simulink model "test_final_sift"  (R2015a)
settings: Solver=ode45  StartTime=0.0  StopTime=10.0  RelTol=1e-3
InitFcn:
  | %% DSPBuilder Start
  | alt_dspbuilder_update_model(bdroot)
  | %% DSPBuilder End
libraries: allblocks_alteradspbuilder2 x2309
(part 5 of 27)

== system test_final_sift/sift_octave1/get_descriptor/hist_bin/Line_buffer_5x5 ==
  dataIn : Inport
  clken : Inport  Port=2
  Delay : allblocks_alteradspbuilder2/Delay  pipeline=1  pipeline_display=1  ClockPhase=1  use_ena=on  use_sclr=off  allowFloatingPointOverride=on  logOutputs=off  logFile=C:\Users\ASUS\Desktop\sift_fpga\Octave_2\tb_test_final_sift\test%5Ffinal%5Fsift_sift%5Foctave1_get%5Fdescriptor_hist%5Fbin_Line%5Fbuffer%5F5x5_Delay.fixedpointlog  use_init=off  reset_value=1
  Delay1 : allblocks_alteradspbuilder2/Delay  pipeline=1  pipeline_display=1  ClockPhase=1  use_ena=on  use_sclr=off  allowFloatingPointOverride=on  logOutputs=off  logFile=C:\Users\ASUS\Desktop\sift_fpga\Octave_2\tb_test_final_sift\test%5Ffinal%5Fsift_sift%5Foctave1_get%5Fdescriptor_hist%5Fbin_Line%5Fbuffer%5F5x5_Delay1.fixedpointlog  use_init=off  reset_value=1
  Delay10 : allblocks_alteradspbuilder2/Delay  pipeline=1  pipeline_display=1  ClockPhase=1  use_ena=on  use_sclr=off  allowFloatingPointOverride=on  logOutputs=off  logFile=C:\Users\ASUS\Desktop\sift_fpga\Octave_2\tb_test_final_sift\test%5Ffinal%5Fsift_sift%5Foctave1_get%5Fdescriptor_hist%5Fbin_Line%5Fbuffer%5F5x5_Delay10.fixedpointlog  use_init=off  reset_value=1
  Delay11 : allblocks_alteradspbuilder2/Delay  pipeline=1  pipeline_display=1  ClockPhase=1  use_ena=on  use_sclr=off  allowFloatingPointOverride=on  logOutputs=off  logFile=C:\Users\ASUS\Desktop\sift_fpga\Octave_2\tb_test_final_sift\test%5Ffinal%5Fsift_sift%5Foctave1_get%5Fdescriptor_hist%5Fbin_Line%5Fbuffer%5F5x5_Delay11.fixedpointlog  use_init=off  reset_value=1
  Delay12 : allblocks_alteradspbuilder2/Delay  pipeline=1  pipeline_display=1  ClockPhase=1  use_ena=on  use_sclr=off  allowFloatingPointOverride=on  logOutputs=off  logFile=C:\Users\ASUS\Desktop\sift_fpga\Octave_2\tb_test_final_sift\test%5Ffinal%5Fsift_sift%5Foctave1_get%5Fdescriptor_hist%5Fbin_Line%5Fbuffer%5F5x5_Delay12.fixedpointlog  use_init=off  reset_value=1
  Delay13 : allblocks_alteradspbuilder2/Delay  pipeline=1  pipeline_display=1  ClockPhase=1  use_ena=on  use_sclr=off  allowFloatingPointOverride=on  logOutputs=off  logFile=C:\Users\ASUS\Desktop\sift_fpga\Octave_2\tb_test_final_sift\test%5Ffinal%5Fsift_sift%5Foctave1_get%5Fdescriptor_hist%5Fbin_Line%5Fbuffer%5F5x5_Delay13.fixedpointlog  use_init=off  reset_value=1
  Delay14 : allblocks_alteradspbuilder2/Delay  pipeline=1  pipeline_display=1  ClockPhase=1  use_ena=on  use_sclr=off  allowFloatingPointOverride=on  logOutputs=off  logFile=C:\Users\ASUS\Desktop\sift_fpga\Octave_2\tb_test_final_sift\test%5Ffinal%5Fsift_sift%5Foctave1_get%5Fdescriptor_hist%5Fbin_Line%5Fbuffer%5F5x5_Delay14.fixedpointlog  use_init=off  reset_value=1
  Delay15 : allblocks_alteradspbuilder2/Delay  pipeline=1  pipeline_display=1  ClockPhase=1  use_ena=on  use_sclr=off  allowFloatingPointOverride=on  logOutputs=off  logFile=C:\Users\ASUS\Desktop\sift_fpga\Octave_2\tb_test_final_sift\test%5Ffinal%5Fsift_sift%5Foctave1_get%5Fdescriptor_hist%5Fbin_Line%5Fbuffer%5F5x5_Delay15.fixedpointlog  use_init=off  reset_value=1
  Delay16 : allblocks_alteradspbuilder2/Delay  pipeline=1  pipeline_display=1  ClockPhase=1  use_ena=on  use_sclr=off  allowFloatingPointOverride=on  logOutputs=off  logFile=C:\Users\ASUS\Desktop\sift_fpga\Octave_2\tb_test_final_sift\test%5Ffinal%5Fsift_sift%5Foctave1_get%5Fdescriptor_hist%5Fbin_Line%5Fbuffer%5F5x5_Delay16.fixedpointlog  use_init=off  reset_value=1
  Delay17 : allblocks_alteradspbuilder2/Delay  pipeline=1  pipeline_display=1  ClockPhase=1  use_ena=on  use_sclr=off  allowFloatingPointOverride=on  logOutputs=off  logFile=C:\Users\ASUS\Desktop\sift_fpga\Octave_2\tb_test_final_sift\test%5Ffinal%5Fsift_sift%5Foctave1_get%5Fdescriptor_hist%5Fbin_Line%5Fbuffer%5F5x5_Delay17.fixedpointlog  use_init=off  reset_value=1
  Delay18 : allblocks_alteradspbuilder2/Delay  pipeline=1  pipeline_display=1  ClockPhase=1  use_ena=on  use_sclr=off  allowFloatingPointOverride=on  logOutputs=off  logFile=C:\Users\ASUS\Desktop\sift_fpga\Octave_2\tb_test_final_sift\test%5Ffinal%5Fsift_sift%5Foctave1_get%5Fdescriptor_hist%5Fbin_Line%5Fbuffer%5F5x5_Delay18.fixedpointlog  use_init=off  reset_value=1
  Delay19 : allblocks_alteradspbuilder2/Delay  pipeline=1  pipeline_display=1  ClockPhase=1  use_ena=on  use_sclr=off  allowFloatingPointOverride=on  logOutputs=off  logFile=C:\Users\ASUS\Desktop\sift_fpga\Octave_2\tb_test_final_sift\test%5Ffinal%5Fsift_sift%5Foctave1_get%5Fdescriptor_hist%5Fbin_Line%5Fbuffer%5F5x5_Delay19.fixedpointlog  use_init=off  reset_value=1
  Delay2 : allblocks_alteradspbuilder2/Delay  pipeline=1  pipeline_display=1  ClockPhase=1  use_ena=on  use_sclr=off  allowFloatingPointOverride=on  logOutputs=off  logFile=C:\Users\ASUS\Desktop\sift_fpga\Octave_2\tb_test_final_sift\test%5Ffinal%5Fsift_sift%5Foctave1_get%5Fdescriptor_hist%5Fbin_Line%5Fbuffer%5F5x5_Delay2.fixedpointlog  use_init=off  reset_value=1
  Delay20 : allblocks_alteradspbuilder2/Delay  pipeline=1  pipeline_display=1  ClockPhase=1  use_ena=on  use_sclr=off  allowFloatingPointOverride=on  logOutputs=off  logFile=C:\Users\ASUS\Desktop\sift_fpga\Octave_2\tb_test_final_sift\test%5Ffinal%5Fsift_sift%5Foctave1_get%5Fdescriptor_hist%5Fbin_Line%5Fbuffer%5F5x5_Delay20.fixedpointlog  use_init=off  reset_value=1
  Delay3 : allblocks_alteradspbuilder2/Delay  pipeline=1  pipeline_display=1  ClockPhase=1  use_ena=on  use_sclr=off  allowFloatingPointOverride=on  logOutputs=off  logFile=C:\Users\ASUS\Desktop\sift_fpga\Octave_2\tb_test_final_sift\test%5Ffinal%5Fsift_sift%5Foctave1_get%5Fdescriptor_hist%5Fbin_Line%5Fbuffer%5F5x5_Delay3.fixedpointlog  use_init=off  reset_value=1
  Delay4 : allblocks_alteradspbuilder2/Delay  pipeline=1  pipeline_display=1  ClockPhase=1  use_ena=on  use_sclr=off  allowFloatingPointOverride=on  logOutputs=off  logFile=C:\Users\ASUS\Desktop\sift_fpga\Octave_2\tb_test_final_sift\test%5Ffinal%5Fsift_sift%5Foctave1_get%5Fdescriptor_hist%5Fbin_Line%5Fbuffer%5F5x5_Delay4.fixedpointlog  use_init=off  reset_value=1
  Delay5 : allblocks_alteradspbuilder2/Delay  pipeline=1  pipeline_display=1  ClockPhase=1  use_ena=on  use_sclr=off  allowFloatingPointOverride=on  logOutputs=off  logFile=C:\Users\ASUS\Desktop\sift_fpga\Octave_2\tb_test_final_sift\test%5Ffinal%5Fsift_sift%5Foctave1_get%5Fdescriptor_hist%5Fbin_Line%5Fbuffer%5F5x5_Delay5.fixedpointlog  use_init=off  reset_value=1
  Delay6 : allblocks_alteradspbuilder2/Delay  pipeline=1  pipeline_display=1  ClockPhase=1  use_ena=on  use_sclr=off  allowFloatingPointOverride=on  logOutputs=off  logFile=C:\Users\ASUS\Desktop\sift_fpga\Octave_2\tb_test_final_sift\test%5Ffinal%5Fsift_sift%5Foctave1_get%5Fdescriptor_hist%5Fbin_Line%5Fbuffer%5F5x5_Delay6.fixedpointlog  use_init=off  reset_value=1
  Delay7 : allblocks_alteradspbuilder2/Delay  pipeline=1  pipeline_display=1  ClockPhase=1  use_ena=on  use_sclr=off  allowFloatingPointOverride=on  logOutputs=off  logFile=C:\Users\ASUS\Desktop\sift_fpga\Octave_2\tb_test_final_sift\test%5Ffinal%5Fsift_sift%5Foctave1_get%5Fdescriptor_hist%5Fbin_Line%5Fbuffer%5F5x5_Delay7.fixedpointlog  use_init=off  reset_value=1
  Delay8 : allblocks_alteradspbuilder2/Delay  pipeline=1  pipeline_display=1  ClockPhase=1  use_ena=on  use_sclr=off  allowFloatingPointOverride=on  logOutputs=off  logFile=C:\Users\ASUS\Desktop\sift_fpga\Octave_2\tb_test_final_sift\test%5Ffinal%5Fsift_sift%5Foctave1_get%5Fdescriptor_hist%5Fbin_Line%5Fbuffer%5F5x5_Delay8.fixedpointlog  use_init=off  reset_value=1
  Delay9 : allblocks_alteradspbuilder2/Delay  pipeline=1  pipeline_display=1  ClockPhase=1  use_ena=on  use_sclr=off  allowFloatingPointOverride=on  logOutputs=off  logFile=C:\Users\ASUS\Desktop\sift_fpga\Octave_2\tb_test_final_sift\test%5Ffinal%5Fsift_sift%5Foctave1_get%5Fdescriptor_hist%5Fbin_Line%5Fbuffer%5F5x5_Delay9.fixedpointlog  use_init=off  reset_value=1
  Memory Delay : allblocks_alteradspbuilder2/Memory Delay  BusType=Unsigned Integer  bwl=10  bwr=0  pipeline=636  pipeline_display=636  ram_type=AUTO  use_ena=on  use_sclr=off  allowFloatingPointOverride=on  logOutputs=off  logFile=C:\Users\ASUS\Desktop\sift_fpga\Octave_2\tb_test_final_sift\test%5Ffinal%5Fsift_sift%5Foctave1_get%5Fdescriptor_hist%5Fbin_Line%5Fbuffer%5F5x5_Memory+Delay.fixedpointlog
  Memory Delay1 : allblocks_alteradspbuilder2/Memory Delay  BusType=Unsigned Integer  bwl=10  bwr=0  pipeline=636  pipeline_display=636  ram_type=AUTO  use_ena=on  use_sclr=off  allowFloatingPointOverride=on  logOutputs=off  logFile=C:\Users\ASUS\Desktop\sift_fpga\Octave_2\tb_test_final_sift\test%5Ffinal%5Fsift_sift%5Foctave1_get%5Fdescriptor_hist%5Fbin_Line%5Fbuffer%5F5x5_Memory+Delay1.fixedpointlog
  Memory Delay2 : allblocks_alteradspbuilder2/Memory Delay  BusType=Unsigned Integer  bwl=10  bwr=0  pipeline=636  pipeline_display=636  ram_type=AUTO  use_ena=on  use_sclr=off  allowFloatingPointOverride=on  logOutputs=off  logFile=C:\Users\ASUS\Desktop\sift_fpga\Octave_2\tb_test_final_sift\test%5Ffinal%5Fsift_sift%5Foctave1_get%5Fdescriptor_hist%5Fbin_Line%5Fbuffer%5F5x5_Memory+Delay2.fixedpointlog
  Memory Delay3 : allblocks_alteradspbuilder2/Memory Delay  BusType=Unsigned Integer  bwl=10  bwr=0  pipeline=636  pipeline_display=636  ram_type=AUTO  use_ena=on  use_sclr=off  allowFloatingPointOverride=on  logOutputs=off  logFile=C:\Users\ASUS\Desktop\sift_fpga\Octave_2\tb_test_final_sift\test%5Ffinal%5Fsift_sift%5Foctave1_get%5Fdescriptor_hist%5Fbin_Line%5Fbuffer%5F5x5_Memory+Delay3.fixedpointlog
  Out00 : Outport
  Out01 : Outport  Port=2
  Out02 : Outport  Port=3
  Out03 : Outport  Port=4
  Out04 : Outport  Port=5
  Out10 : Outport  Port=6
  Out11 : Outport  Port=7
  Out12 : Outport  Port=8
  Out13 : Outport  Port=9
  Out14 : Outport  Port=10
  Out20 : Outport  Port=11
  Out21 : Outport  Port=12
  Out22 : Outport  Port=13
  Out23 : Outport  Port=14
  Out24 : Outport  Port=15
  Out30 : Outport  Port=16
  Out31 : Outport  Port=17
  Out32 : Outport  Port=18
  Out33 : Outport  Port=19
  Out34 : Outport  Port=20
  Out40 : Outport  Port=21
  Out41 : Outport  Port=22
  Out42 : Outport  Port=23
  Out43 : Outport  Port=24
  Out44 : Outport  Port=25
  wires:
  [clken] -> Delay11/2
  Delay11/1 -> [data_23], Delay12/1
  [clken] -> Delay12/2
  [clken] -> Delay10/2
  Delay8/1 -> Memory Delay1/1, [data_14]
  [clken] -> Memory Delay1/2
  Delay9/1 -> [data_21], Delay10/1
  Memory Delay1/1 -> [data_20], Delay9/1
  Delay10/1 -> [data_22], Delay11/1
  [clken] -> Delay9/2
  [clken] -> Delay4/2
  [data_03] -> Out03/1
  [data_04] -> Out04/1
  [data_02] -> Out02/1
  Delay/1 -> [data_00], Delay1/1
  [data_32] -> Out32/1
  [data_44] -> Out44/1
  [data_31] -> Out31/1
  [data_40] -> Out40/1
  [data_34] -> Out34/1
  [data_30] -> Out30/1
  [data_33] -> Out33/1
  [data_43] -> Out43/1
  [data_42] -> Out42/1
  [data_41] -> Out41/1
  [clken] -> Delay1/2
  [clken] -> Delay/2
  [data_in] -> Delay/1
  [clken] -> Delay2/2
  Delay2/1 -> [data_02], Delay3/1
  Delay1/1 -> [data_01], Delay2/1
  [clken] -> Delay3/2
  [data_01] -> Out01/1
  clken/1 -> [clken]
  [data_00] -> Out00/1
  [data_21] -> Out21/1
  [data_20] -> Out20/1
  [data_23] -> Out23/1
  [data_22] -> Out22/1
  [data_24] -> Out24/1
  dataIn/1 -> [data_in]
  [data_10] -> Out10/1
  [data_11] -> Out11/1
  [data_12] -> Out12/1
  [data_13] -> Out13/1
  [data_14] -> Out14/1
  Delay4/1 -> Memory Delay/1, [data_04]
  [clken] -> Memory Delay/2
  Delay12/1 -> [data_24], Memory Delay2/1
  [clken] -> Memory Delay2/2
  Memory Delay2/1 -> [data_30], Delay16/1
  [clken] -> Delay16/2
  [clken] -> Delay14/2
  [clken] -> Delay15/2
  [clken] -> Memory Delay3/2
  Delay17/1 -> [data_32], Delay18/1
  Delay18/1 -> [data_33], Delay19/1
  Memory Delay3/1 -> [data_40], Delay20/1
  [clken] -> Delay20/2
  [clken] -> Delay19/2
  Delay13/1 -> [data_42], Delay14/1
  Delay19/1 -> Memory Delay3/1, [data_34]
  Delay14/1 -> [data_43], Delay15/1
  Delay15/1 -> [data_44]
  [clken] -> Delay17/2
  [clken] -> Delay18/2
  [clken] -> Delay13/2
  Delay16/1 -> [data_31], Delay17/1
  Delay20/1 -> [data_41], Delay13/1
  Memory Delay/1 -> [data_10], Delay5/1
  [clken] -> Delay7/2
  [clken] -> Delay6/2
  Delay5/1 -> [data_11], Delay6/1
  [clken] -> Delay8/2
  [clken] -> Delay5/2
  Delay7/1 -> [data_13], Delay8/1
  Delay6/1 -> [data_12], Delay7/1
  Delay3/1 -> [data_03], Delay4/1

== system test_final_sift/sift_octave1/get_descriptor/hist_bin/Line_buffer_5x5_1 ==
  dataIn : Inport
  clken : Inport  Port=2
  Delay : allblocks_alteradspbuilder2/Delay  pipeline=1  pipeline_display=1  ClockPhase=1  use_ena=on  use_sclr=off  allowFloatingPointOverride=on  logOutputs=off  logFile=C:\Users\ASUS\Desktop\sift_fpga\Octave_2\tb_test_final_sift\test%5Ffinal%5Fsift_sift%5Foctave1_get%5Fdescriptor_hist%5Fbin_Line%5Fbuffer%5F5x5%5F1_Delay.fixedpointlog  use_init=off  reset_value=1
  Delay1 : allblocks_alteradspbuilder2/Delay  pipeline=1  pipeline_display=1  ClockPhase=1  use_ena=on  use_sclr=off  allowFloatingPointOverride=on  logOutputs=off  logFile=C:\Users\ASUS\Desktop\sift_fpga\Octave_2\tb_test_final_sift\test%5Ffinal%5Fsift_sift%5Foctave1_get%5Fdescriptor_hist%5Fbin_Line%5Fbuffer%5F5x5%5F1_Delay1.fixedpointlog  use_init=off  reset_value=1
  Delay10 : allblocks_alteradspbuilder2/Delay  pipeline=1  pipeline_display=1  ClockPhase=1  use_ena=on  use_sclr=off  allowFloatingPointOverride=on  logOutputs=off  logFile=C:\Users\ASUS\Desktop\sift_fpga\Octave_2\tb_test_final_sift\test%5Ffinal%5Fsift_sift%5Foctave1_get%5Fdescriptor_hist%5Fbin_Line%5Fbuffer%5F5x5%5F1_Delay10.fixedpointlog  use_init=off  reset_value=1
  Delay11 : allblocks_alteradspbuilder2/Delay  pipeline=1  pipeline_display=1  ClockPhase=1  use_ena=on  use_sclr=off  allowFloatingPointOverride=on  logOutputs=off  logFile=C:\Users\ASUS\Desktop\sift_fpga\Octave_2\tb_test_final_sift\test%5Ffinal%5Fsift_sift%5Foctave1_get%5Fdescriptor_hist%5Fbin_Line%5Fbuffer%5F5x5%5F1_Delay11.fixedpointlog  use_init=off  reset_value=1
  Delay12 : allblocks_alteradspbuilder2/Delay  pipeline=1  pipeline_display=1  ClockPhase=1  use_ena=on  use_sclr=off  allowFloatingPointOverride=on  logOutputs=off  logFile=C:\Users\ASUS\Desktop\sift_fpga\Octave_2\tb_test_final_sift\test%5Ffinal%5Fsift_sift%5Foctave1_get%5Fdescriptor_hist%5Fbin_Line%5Fbuffer%5F5x5%5F1_Delay12.fixedpointlog  use_init=off  reset_value=1
  Delay13 : allblocks_alteradspbuilder2/Delay  pipeline=1  pipeline_display=1  ClockPhase=1  use_ena=on  use_sclr=off  allowFloatingPointOverride=on  logOutputs=off  logFile=C:\Users\ASUS\Desktop\sift_fpga\Octave_2\tb_test_final_sift\test%5Ffinal%5Fsift_sift%5Foctave1_get%5Fdescriptor_hist%5Fbin_Line%5Fbuffer%5F5x5%5F1_Delay13.fixedpointlog  use_init=off  reset_value=1
  Delay14 : allblocks_alteradspbuilder2/Delay  pipeline=1  pipeline_display=1  ClockPhase=1  use_ena=on  use_sclr=off  allowFloatingPointOverride=on  logOutputs=off  logFile=C:\Users\ASUS\Desktop\sift_fpga\Octave_2\tb_test_final_sift\test%5Ffinal%5Fsift_sift%5Foctave1_get%5Fdescriptor_hist%5Fbin_Line%5Fbuffer%5F5x5%5F1_Delay14.fixedpointlog  use_init=off  reset_value=1
  Delay15 : allblocks_alteradspbuilder2/Delay  pipeline=1  pipeline_display=1  ClockPhase=1  use_ena=on  use_sclr=off  allowFloatingPointOverride=on  logOutputs=off  logFile=C:\Users\ASUS\Desktop\sift_fpga\Octave_2\tb_test_final_sift\test%5Ffinal%5Fsift_sift%5Foctave1_get%5Fdescriptor_hist%5Fbin_Line%5Fbuffer%5F5x5%5F1_Delay15.fixedpointlog  use_init=off  reset_value=1
  Delay16 : allblocks_alteradspbuilder2/Delay  pipeline=1  pipeline_display=1  ClockPhase=1  use_ena=on  use_sclr=off  allowFloatingPointOverride=on  logOutputs=off  logFile=C:\Users\ASUS\Desktop\sift_fpga\Octave_2\tb_test_final_sift\test%5Ffinal%5Fsift_sift%5Foctave1_get%5Fdescriptor_hist%5Fbin_Line%5Fbuffer%5F5x5%5F1_Delay16.fixedpointlog  use_init=off  reset_value=1
  Delay17 : allblocks_alteradspbuilder2/Delay  pipeline=1  pipeline_display=1  ClockPhase=1  use_ena=on  use_sclr=off  allowFloatingPointOverride=on  logOutputs=off  logFile=C:\Users\ASUS\Desktop\sift_fpga\Octave_2\tb_test_final_sift\test%5Ffinal%5Fsift_sift%5Foctave1_get%5Fdescriptor_hist%5Fbin_Line%5Fbuffer%5F5x5%5F1_Delay17.fixedpointlog  use_init=off  reset_value=1
  Delay18 : allblocks_alteradspbuilder2/Delay  pipeline=1  pipeline_display=1  ClockPhase=1  use_ena=on  use_sclr=off  allowFloatingPointOverride=on  logOutputs=off  logFile=C:\Users\ASUS\Desktop\sift_fpga\Octave_2\tb_test_final_sift\test%5Ffinal%5Fsift_sift%5Foctave1_get%5Fdescriptor_hist%5Fbin_Line%5Fbuffer%5F5x5%5F1_Delay18.fixedpointlog  use_init=off  reset_value=1
  Delay19 : allblocks_alteradspbuilder2/Delay  pipeline=1  pipeline_display=1  ClockPhase=1  use_ena=on  use_sclr=off  allowFloatingPointOverride=on  logOutputs=off  logFile=C:\Users\ASUS\Desktop\sift_fpga\Octave_2\tb_test_final_sift\test%5Ffinal%5Fsift_sift%5Foctave1_get%5Fdescriptor_hist%5Fbin_Line%5Fbuffer%5F5x5%5F1_Delay19.fixedpointlog  use_init=off  reset_value=1
  Delay2 : allblocks_alteradspbuilder2/Delay  pipeline=1  pipeline_display=1  ClockPhase=1  use_ena=on  use_sclr=off  allowFloatingPointOverride=on  logOutputs=off  logFile=C:\Users\ASUS\Desktop\sift_fpga\Octave_2\tb_test_final_sift\test%5Ffinal%5Fsift_sift%5Foctave1_get%5Fdescriptor_hist%5Fbin_Line%5Fbuffer%5F5x5%5F1_Delay2.fixedpointlog  use_init=off  reset_value=1
  Delay20 : allblocks_alteradspbuilder2/Delay  pipeline=1  pipeline_display=1  ClockPhase=1  use_ena=on  use_sclr=off  allowFloatingPointOverride=on  logOutputs=off  logFile=C:\Users\ASUS\Desktop\sift_fpga\Octave_2\tb_test_final_sift\test%5Ffinal%5Fsift_sift%5Foctave1_get%5Fdescriptor_hist%5Fbin_Line%5Fbuffer%5F5x5%5F1_Delay20.fixedpointlog  use_init=off  reset_value=1
  Delay3 : allblocks_alteradspbuilder2/Delay  pipeline=1  pipeline_display=1  ClockPhase=1  use_ena=on  use_sclr=off  allowFloatingPointOverride=on  logOutputs=off  logFile=C:\Users\ASUS\Desktop\sift_fpga\Octave_2\tb_test_final_sift\test%5Ffinal%5Fsift_sift%5Foctave1_get%5Fdescriptor_hist%5Fbin_Line%5Fbuffer%5F5x5%5F1_Delay3.fixedpointlog  use_init=off  reset_value=1
  Delay4 : allblocks_alteradspbuilder2/Delay  pipeline=1  pipeline_display=1  ClockPhase=1  use_ena=on  use_sclr=off  allowFloatingPointOverride=on  logOutputs=off  logFile=C:\Users\ASUS\Desktop\sift_fpga\Octave_2\tb_test_final_sift\test%5Ffinal%5Fsift_sift%5Foctave1_get%5Fdescriptor_hist%5Fbin_Line%5Fbuffer%5F5x5%5F1_Delay4.fixedpointlog  use_init=off  reset_value=1
  Delay5 : allblocks_alteradspbuilder2/Delay  pipeline=1  pipeline_display=1  ClockPhase=1  use_ena=on  use_sclr=off  allowFloatingPointOverride=on  logOutputs=off  logFile=C:\Users\ASUS\Desktop\sift_fpga\Octave_2\tb_test_final_sift\test%5Ffinal%5Fsift_sift%5Foctave1_get%5Fdescriptor_hist%5Fbin_Line%5Fbuffer%5F5x5%5F1_Delay5.fixedpointlog  use_init=off  reset_value=1
  Delay6 : allblocks_alteradspbuilder2/Delay  pipeline=1  pipeline_display=1  ClockPhase=1  use_ena=on  use_sclr=off  allowFloatingPointOverride=on  logOutputs=off  logFile=C:\Users\ASUS\Desktop\sift_fpga\Octave_2\tb_test_final_sift\test%5Ffinal%5Fsift_sift%5Foctave1_get%5Fdescriptor_hist%5Fbin_Line%5Fbuffer%5F5x5%5F1_Delay6.fixedpointlog  use_init=off  reset_value=1
  Delay7 : allblocks_alteradspbuilder2/Delay  pipeline=1  pipeline_display=1  ClockPhase=1  use_ena=on  use_sclr=off  allowFloatingPointOverride=on  logOutputs=off  logFile=C:\Users\ASUS\Desktop\sift_fpga\Octave_2\tb_test_final_sift\test%5Ffinal%5Fsift_sift%5Foctave1_get%5Fdescriptor_hist%5Fbin_Line%5Fbuffer%5F5x5%5F1_Delay7.fixedpointlog  use_init=off  reset_value=1
  Delay8 : allblocks_alteradspbuilder2/Delay  pipeline=1  pipeline_display=1  ClockPhase=1  use_ena=on  use_sclr=off  allowFloatingPointOverride=on  logOutputs=off  logFile=C:\Users\ASUS\Desktop\sift_fpga\Octave_2\tb_test_final_sift\test%5Ffinal%5Fsift_sift%5Foctave1_get%5Fdescriptor_hist%5Fbin_Line%5Fbuffer%5F5x5%5F1_Delay8.fixedpointlog  use_init=off  reset_value=1
  Delay9 : allblocks_alteradspbuilder2/Delay  pipeline=1  pipeline_display=1  ClockPhase=1  use_ena=on  use_sclr=off  allowFloatingPointOverride=on  logOutputs=off  logFile=C:\Users\ASUS\Desktop\sift_fpga\Octave_2\tb_test_final_sift\test%5Ffinal%5Fsift_sift%5Foctave1_get%5Fdescriptor_hist%5Fbin_Line%5Fbuffer%5F5x5%5F1_Delay9.fixedpointlog  use_init=off  reset_value=1
  Memory Delay : allblocks_alteradspbuilder2/Memory Delay  BusType=Unsigned Integer  bwl=8  bwr=0  pipeline=636  pipeline_display=636  ram_type=AUTO  use_ena=on  use_sclr=off  allowFloatingPointOverride=on  logOutputs=off  logFile=C:\Users\ASUS\Desktop\sift_fpga\Octave_2\tb_test_final_sift\test%5Ffinal%5Fsift_sift%5Foctave1_get%5Fdescriptor_hist%5Fbin_Line%5Fbuffer%5F5x5%5F1_Memory+Delay.fixedpointlog
  Memory Delay1 : allblocks_alteradspbuilder2/Memory Delay  BusType=Unsigned Integer  bwl=8  bwr=0  pipeline=636  pipeline_display=636  ram_type=AUTO  use_ena=on  use_sclr=off  allowFloatingPointOverride=on  logOutputs=off  logFile=C:\Users\ASUS\Desktop\sift_fpga\Octave_2\tb_test_final_sift\test%5Ffinal%5Fsift_sift%5Foctave1_get%5Fdescriptor_hist%5Fbin_Line%5Fbuffer%5F5x5%5F1_Memory+Delay1.fixedpointlog
  Memory Delay2 : allblocks_alteradspbuilder2/Memory Delay  BusType=Unsigned Integer  bwl=8  bwr=0  pipeline=636  pipeline_display=636  ram_type=AUTO  use_ena=on  use_sclr=off  allowFloatingPointOverride=on  logOutputs=off  logFile=C:\Users\ASUS\Desktop\sift_fpga\Octave_2\tb_test_final_sift\test%5Ffinal%5Fsift_sift%5Foctave1_get%5Fdescriptor_hist%5Fbin_Line%5Fbuffer%5F5x5%5F1_Memory+Delay2.fixedpointlog
  Memory Delay3 : allblocks_alteradspbuilder2/Memory Delay  BusType=Unsigned Integer  bwl=8  bwr=0  pipeline=636  pipeline_display=636  ram_type=AUTO  use_ena=on  use_sclr=off  allowFloatingPointOverride=on  logOutputs=off  logFile=C:\Users\ASUS\Desktop\sift_fpga\Octave_2\tb_test_final_sift\test%5Ffinal%5Fsift_sift%5Foctave1_get%5Fdescriptor_hist%5Fbin_Line%5Fbuffer%5F5x5%5F1_Memory+Delay3.fixedpointlog
  Out00 : Outport
  Out01 : Outport  Port=2
  Out02 : Outport  Port=3
  Out03 : Outport  Port=4
  Out04 : Outport  Port=5
  Out10 : Outport  Port=6
  Out11 : Outport  Port=7
  Out12 : Outport  Port=8
  Out13 : Outport  Port=9
  Out14 : Outport  Port=10
  Out20 : Outport  Port=11
  Out21 : Outport  Port=12
  Out22 : Outport  Port=13
  Out23 : Outport  Port=14
  Out24 : Outport  Port=15
  Out30 : Outport  Port=16
  Out31 : Outport  Port=17
  Out32 : Outport  Port=18
  Out33 : Outport  Port=19
  Out34 : Outport  Port=20
  Out40 : Outport  Port=21
  Out41 : Outport  Port=22
  Out42 : Outport  Port=23
  Out43 : Outport  Port=24
  Out44 : Outport  Port=25
  wires:
  [clken] -> Delay11/2
  Delay11/1 -> [data_23], Delay12/1
  [clken] -> Delay12/2
  [clken] -> Delay10/2
  Delay8/1 -> Memory Delay1/1, [data_14]
  [clken] -> Memory Delay1/2
  Delay9/1 -> [data_21], Delay10/1
  Memory Delay1/1 -> [data_20], Delay9/1
  Delay10/1 -> [data_22], Delay11/1
  [clken] -> Delay9/2
  [clken] -> Delay4/2
  [data_03] -> Out03/1
  [data_04] -> Out04/1
  [data_02] -> Out02/1
  Delay/1 -> [data_00], Delay1/1
  [data_32] -> Out32/1
  [data_44] -> Out44/1
  [data_31] -> Out31/1
  [data_40] -> Out40/1
  [data_34] -> Out34/1
  [data_30] -> Out30/1
  [data_33] -> Out33/1
  [data_43] -> Out43/1
  [data_42] -> Out42/1
  [data_41] -> Out41/1
  [clken] -> Delay1/2
  [clken] -> Delay/2
  [data_in] -> Delay/1
  [clken] -> Delay2/2
  Delay2/1 -> [data_02], Delay3/1
  Delay1/1 -> [data_01], Delay2/1
  [clken] -> Delay3/2
  [data_01] -> Out01/1
  clken/1 -> [clken]
  [data_00] -> Out00/1
  [data_21] -> Out21/1
  [data_20] -> Out20/1
  [data_23] -> Out23/1
  [data_22] -> Out22/1
  [data_24] -> Out24/1
  dataIn/1 -> [data_in]
  [data_10] -> Out10/1
  [data_11] -> Out11/1
  [data_12] -> Out12/1
  [data_13] -> Out13/1
  [data_14] -> Out14/1
  Delay4/1 -> Memory Delay/1, [data_04]
  [clken] -> Memory Delay/2
  Delay12/1 -> [data_24], Memory Delay2/1
  [clken] -> Memory Delay2/2
  Memory Delay2/1 -> [data_30], Delay16/1
  [clken] -> Delay16/2
  [clken] -> Delay14/2
  [clken] -> Delay15/2
  [clken] -> Memory Delay3/2
  Delay17/1 -> [data_32], Delay18/1
  Delay18/1 -> [data_33], Delay19/1
  Memory Delay3/1 -> [data_40], Delay20/1
  [clken] -> Delay20/2
  [clken] -> Delay19/2
  Delay13/1 -> [data_42], Delay14/1
  Delay19/1 -> Memory Delay3/1, [data_34]
  Delay14/1 -> [data_43], Delay15/1
  Delay15/1 -> [data_44]
  [clken] -> Delay17/2
  [clken] -> Delay18/2
  [clken] -> Delay13/2
  Delay16/1 -> [data_31], Delay17/1
  Delay20/1 -> [data_41], Delay13/1
  Memory Delay/1 -> [data_10], Delay5/1
  [clken] -> Delay7/2
  [clken] -> Delay6/2
  Delay5/1 -> [data_11], Delay6/1
  [clken] -> Delay8/2
  [clken] -> Delay5/2
  Delay7/1 -> [data_13], Delay8/1
  Delay6/1 -> [data_12], Delay7/1
  Delay3/1 -> [data_03], Delay4/1

== system test_final_sift/sift_octave1/get_descriptor/hist_bin/Subsystem ==
  hist_in_bin1 : Inport
  hist_in_bin2 : Inport  Port=2
  hist_in_bin3 : Inport  Port=3
  hist_in_bin4 : Inport  Port=4
  hist_in_bin5 : Inport  Port=5
  hist_in_bin6 : Inport  Port=6
  hist_in_bin7 : Inport  Port=7
  hist_in_bin8 : Inport  Port=8
  Comparator1 : allblocks_alteradspbuilder2/Comparator  direction=a < b  pipeline_display=0  allowFloatingPointOverride=on  logOutputs=off  logFile=C:\Users\ASUS\Desktop\sift_fpga\Octave_2\tb_test_final_sift\test%5Ffinal%5Fsift_sift%5Foctave1_get%5Fdescriptor_hist%5Fbin_Subsystem_Comparator1.fixedpointlog
  Comparator10 : allblocks_alteradspbuilder2/Comparator  direction=a < b  pipeline_display=0  allowFloatingPointOverride=on  logOutputs=off  logFile=C:\Users\ASUS\Desktop\sift_fpga\Octave_2\tb_test_final_sift\test%5Ffinal%5Fsift_sift%5Foctave1_get%5Fdescriptor_hist%5Fbin_Subsystem_Comparator10.fixedpointlog
  Comparator11 : allblocks_alteradspbuilder2/Comparator  direction=a < b  pipeline_display=0  allowFloatingPointOverride=on  logOutputs=off  logFile=C:\Users\ASUS\Desktop\sift_fpga\Octave_2\tb_test_final_sift\test%5Ffinal%5Fsift_sift%5Foctave1_get%5Fdescriptor_hist%5Fbin_Subsystem_Comparator11.fixedpointlog
  Comparator12 : allblocks_alteradspbuilder2/Comparator  direction=a < b  pipeline_display=0  allowFloatingPointOverride=on  logOutputs=off  logFile=C:\Users\ASUS\Desktop\sift_fpga\Octave_2\tb_test_final_sift\test%5Ffinal%5Fsift_sift%5Foctave1_get%5Fdescriptor_hist%5Fbin_Subsystem_Comparator12.fixedpointlog
  Comparator13 : allblocks_alteradspbuilder2/Comparator  direction=a < b  pipeline_display=0  allowFloatingPointOverride=on  logOutputs=off  logFile=C:\Users\ASUS\Desktop\sift_fpga\Octave_2\tb_test_final_sift\test%5Ffinal%5Fsift_sift%5Foctave1_get%5Fdescriptor_hist%5Fbin_Subsystem_Comparator13.fixedpointlog
  Comparator14 : allblocks_alteradspbuilder2/Comparator  direction=a < b  pipeline_display=0  allowFloatingPointOverride=on  logOutputs=off  logFile=C:\Users\ASUS\Desktop\sift_fpga\Octave_2\tb_test_final_sift\test%5Ffinal%5Fsift_sift%5Foctave1_get%5Fdescriptor_hist%5Fbin_Subsystem_Comparator14.fixedpointlog
  Comparator19 : allblocks_alteradspbuilder2/Comparator  direction=a < b  pipeline_display=0  allowFloatingPointOverride=on  logOutputs=off  logFile=C:\Users\ASUS\Desktop\sift_fpga\Octave_2\tb_test_final_sift\test%5Ffinal%5Fsift_sift%5Foctave1_get%5Fdescriptor_hist%5Fbin_Subsystem_Comparator19.fixedpointlog
  Comparator2 : allblocks_alteradspbuilder2/Comparator  direction=a < b  pipeline_display=0  allowFloatingPointOverride=on  logOutputs=off  logFile=C:\Users\ASUS\Desktop\sift_fpga\Octave_2\tb_test_final_sift\test%5Ffinal%5Fsift_sift%5Foctave1_get%5Fdescriptor_hist%5Fbin_Subsystem_Comparator2.fixedpointlog
  Comparator3 : allblocks_alteradspbuilder2/Comparator  direction=a < b  pipeline_display=0  allowFloatingPointOverride=on  logOutputs=off  logFile=C:\Users\ASUS\Desktop\sift_fpga\Octave_2\tb_test_final_sift\test%5Ffinal%5Fsift_sift%5Foctave1_get%5Fdescriptor_hist%5Fbin_Subsystem_Comparator3.fixedpointlog
  Comparator4 : allblocks_alteradspbuilder2/Comparator  direction=a < b  pipeline_display=0  allowFloatingPointOverride=on  logOutputs=off  logFile=C:\Users\ASUS\Desktop\sift_fpga\Octave_2\tb_test_final_sift\test%5Ffinal%5Fsift_sift%5Foctave1_get%5Fdescriptor_hist%5Fbin_Subsystem_Comparator4.fixedpointlog
  Comparator5 : allblocks_alteradspbuilder2/Comparator  direction=a < b  pipeline_display=0  allowFloatingPointOverride=on  logOutputs=off  logFile=C:\Users\ASUS\Desktop\sift_fpga\Octave_2\tb_test_final_sift\test%5Ffinal%5Fsift_sift%5Foctave1_get%5Fdescriptor_hist%5Fbin_Subsystem_Comparator5.fixedpointlog
  Comparator6 : allblocks_alteradspbuilder2/Comparator  direction=a < b  pipeline_display=0  allowFloatingPointOverride=on  logOutputs=off  logFile=C:\Users\ASUS\Desktop\sift_fpga\Octave_2\tb_test_final_sift\test%5Ffinal%5Fsift_sift%5Foctave1_get%5Fdescriptor_hist%5Fbin_Subsystem_Comparator6.fixedpointlog
  Comparator7 : allblocks_alteradspbuilder2/Comparator  direction=a < b  pipeline_display=0  allowFloatingPointOverride=on  logOutputs=off  logFile=C:\Users\ASUS\Desktop\sift_fpga\Octave_2\tb_test_final_sift\test%5Ffinal%5Fsift_sift%5Foctave1_get%5Fdescriptor_hist%5Fbin_Subsystem_Comparator7.fixedpointlog
  Comparator8 : allblocks_alteradspbuilder2/Comparator  direction=a < b  pipeline_display=0  allowFloatingPointOverride=on  logOutputs=off  logFile=C:\Users\ASUS\Desktop\sift_fpga\Octave_2\tb_test_final_sift\test%5Ffinal%5Fsift_sift%5Foctave1_get%5Fdescriptor_hist%5Fbin_Subsystem_Comparator8.fixedpointlog
  Comparator9 : allblocks_alteradspbuilder2/Comparator  direction=a < b  pipeline_display=0  allowFloatingPointOverride=on  logOutputs=off  logFile=C:\Users\ASUS\Desktop\sift_fpga\Octave_2\tb_test_final_sift\test%5Ffinal%5Fsift_sift%5Foctave1_get%5Fdescriptor_hist%5Fbin_Subsystem_Comparator9.fixedpointlog
  Constant : allblocks_alteradspbuilder2/Constant  mask_cst=0  BusType=Unsigned Integer  bwl=16  bwr=0  roundMode=Truncate  satMode=Wrap  SpecifyClock=off  allowFloatingPointOverride=on  logOutputs=off  logFile=C:\Users\ASUS\Desktop\sift_fpga\Octave_2\tb_test_final_sift\test%5Ffinal%5Fsift_sift%5Foctave1_get%5Fdescriptor_hist%5Fbin_Subsystem_Constant.fixedpointlog
  Constant1 : allblocks_alteradspbuilder2/Constant  mask_cst=0  BusType=Unsigned Integer  bwl=16  bwr=0  roundMode=Truncate  satMode=Wrap  SpecifyClock=off  allowFloatingPointOverride=on  logOutputs=off  logFile=C:\Users\ASUS\Desktop\sift_fpga\Octave_2\tb_test_final_sift\test%5Ffinal%5Fsift_sift%5Foctave1_get%5Fdescriptor_hist%5Fbin_Subsystem_Constant1.fixedpointlog
  Constant2 : allblocks_alteradspbuilder2/Constant  mask_cst=0  BusType=Unsigned Integer  bwl=16  bwr=0  roundMode=Truncate  satMode=Wrap  SpecifyClock=off  allowFloatingPointOverride=on  logOutputs=off  logFile=C:\Users\ASUS\Desktop\sift_fpga\Octave_2\tb_test_final_sift\test%5Ffinal%5Fsift_sift%5Foctave1_get%5Fdescriptor_hist%5Fbin_Subsystem_Constant2.fixedpointlog
  Constant3 : allblocks_alteradspbuilder2/Constant  mask_cst=0  BusType=Unsigned Integer  bwl=16  bwr=0  roundMode=Truncate  satMode=Wrap  SpecifyClock=off  allowFloatingPointOverride=on  logOutputs=off  logFile=C:\Users\ASUS\Desktop\sift_fpga\Octave_2\tb_test_final_sift\test%5Ffinal%5Fsift_sift%5Foctave1_get%5Fdescriptor_hist%5Fbin_Subsystem_Constant3.fixedpointlog
  Constant4 : allblocks_alteradspbuilder2/Constant  mask_cst=0  BusType=Unsigned Integer  bwl=16  bwr=0  roundMode=Truncate  satMode=Wrap  SpecifyClock=off  allowFloatingPointOverride=on  logOutputs=off  logFile=C:\Users\ASUS\Desktop\sift_fpga\Octave_2\tb_test_final_sift\test%5Ffinal%5Fsift_sift%5Foctave1_get%5Fdescriptor_hist%5Fbin_Subsystem_Constant4.fixedpointlog
  Constant5 : allblocks_alteradspbuilder2/Constant  mask_cst=0  BusType=Unsigned Integer  bwl=16  bwr=0  roundMode=Truncate  satMode=Wrap  SpecifyClock=off  allowFloatingPointOverride=on  logOutputs=off  logFile=C:\Users\ASUS\Desktop\sift_fpga\Octave_2\tb_test_final_sift\test%5Ffinal%5Fsift_sift%5Foctave1_get%5Fdescriptor_hist%5Fbin_Subsystem_Constant5.fixedpointlog
  Constant6 : allblocks_alteradspbuilder2/Constant  mask_cst=0  BusType=Unsigned Integer  bwl=8  bwr=0  roundMode=Truncate  satMode=Wrap  SpecifyClock=off  allowFloatingPointOverride=on  logOutputs=off  logFile=C:\Users\ASUS\Desktop\sift_fpga\Octave_2\tb_test_final_sift\test%5Ffinal%5Fsift_sift%5Foctave1_get%5Fdescriptor_hist%5Fbin_Subsystem_Constant6.fixedpointlog
  Constant7 : allblocks_alteradspbuilder2/Constant  mask_cst=0  BusType=Unsigned Integer  bwl=16  bwr=0  roundMode=Truncate  satMode=Wrap  SpecifyClock=off  allowFloatingPointOverride=on  logOutputs=off  logFile=C:\Users\ASUS\Desktop\sift_fpga\Octave_2\tb_test_final_sift\test%5Ffinal%5Fsift_sift%5Foctave1_get%5Fdescriptor_hist%5Fbin_Subsystem_Constant7.fixedpointlog
  Logical Bus Operator : allblocks_alteradspbuilder2/Logical Bus Operator  BusType=Unsigned Integer  bwl=16  bwr=0  LogicalOp_text=Shift Right  mask_value_num=-5  shift_amount=3  force_sign_ext=off  pipeline_display=0
  Multiplexer1 : allblocks_alteradspbuilder2/Multiplexer  numInputs=2  pipeline=0  oneHot=off  pipeline_display=0  use_ena=off  use_aclr=off  allowFloatingPointOverride=on  logOutputs=off  logFile=C:\Users\ASUS\Desktop\sift_fpga\Octave_2\tb_test_final_sift\test%5Ffinal%5Fsift_sift%5Foctave1_get%5Fdescriptor_hist%5Fbin_Subsystem_Multiplexer1.fixedpointlog
  Multiplexer10 : allblocks_alteradspbuilder2/Multiplexer  numInputs=2  pipeline=0  oneHot=off  pipeline_display=0  use_ena=off  use_aclr=off  allowFloatingPointOverride=on  logOutputs=off  logFile=C:\Users\ASUS\Desktop\sift_fpga\Octave_2\tb_test_final_sift\test%5Ffinal%5Fsift_sift%5Foctave1_get%5Fdescriptor_hist%5Fbin_Subsystem_Multiplexer10.fixedpointlog
  Multiplexer11 : allblocks_alteradspbuilder2/Multiplexer  numInputs=2  pipeline=0  oneHot=off  pipeline_display=0  use_ena=off  use_aclr=off  allowFloatingPointOverride=on  logOutputs=off  logFile=C:\Users\ASUS\Desktop\sift_fpga\Octave_2\tb_test_final_sift\test%5Ffinal%5Fsift_sift%5Foctave1_get%5Fdescriptor_hist%5Fbin_Subsystem_Multiplexer11.fixedpointlog
  Multiplexer12 : allblocks_alteradspbuilder2/Multiplexer  numInputs=2  pipeline=0  oneHot=off  pipeline_display=0  use_ena=off  use_aclr=off  allowFloatingPointOverride=on  logOutputs=off  logFile=C:\Users\ASUS\Desktop\sift_fpga\Octave_2\tb_test_final_sift\test%5Ffinal%5Fsift_sift%5Foctave1_get%5Fdescriptor_hist%5Fbin_Subsystem_Multiplexer12.fixedpointlog
  Multiplexer13 : allblocks_alteradspbuilder2/Multiplexer  numInputs=2  pipeline=0  oneHot=off  pipeline_display=0  use_ena=off  use_aclr=off  allowFloatingPointOverride=on  logOutputs=off  logFile=C:\Users\ASUS\Desktop\sift_fpga\Octave_2\tb_test_final_sift\test%5Ffinal%5Fsift_sift%5Foctave1_get%5Fdescriptor_hist%5Fbin_Subsystem_Multiplexer13.fixedpointlog
  Multiplexer14 : allblocks_alteradspbuilder2/Multiplexer  numInputs=2  pipeline=0  oneHot=off  pipeline_display=0  use_ena=off  use_aclr=off  allowFloatingPointOverride=on  logOutputs=off  logFile=C:\Users\ASUS\Desktop\sift_fpga\Octave_2\tb_test_final_sift\test%5Ffinal%5Fsift_sift%5Foctave1_get%5Fdescriptor_hist%5Fbin_Subsystem_Multiplexer14.fixedpointlog
  Multiplexer2 : allblocks_alteradspbuilder2/Multiplexer  numInputs=2  pipeline=0  oneHot=off  pipeline_display=0  use_ena=off  use_aclr=off  allowFloatingPointOverride=on  logOutputs=off  logFile=C:\Users\ASUS\Desktop\sift_fpga\Octave_2\tb_test_final_sift\test%5Ffinal%5Fsift_sift%5Foctave1_get%5Fdescriptor_hist%5Fbin_Subsystem_Multiplexer2.fixedpointlog
  Multiplexer20 : allblocks_alteradspbuilder2/Multiplexer  numInputs=2  pipeline=0  oneHot=off  pipeline_display=0  use_ena=off  use_aclr=off  allowFloatingPointOverride=on  logOutputs=off  logFile=C:\Users\ASUS\Desktop\sift_fpga\Octave_2\tb_test_final_sift\test%5Ffinal%5Fsift_sift%5Foctave1_get%5Fdescriptor_hist%5Fbin_Subsystem_Multiplexer20.fixedpointlog
  Multiplexer3 : allblocks_alteradspbuilder2/Multiplexer  numInputs=2  pipeline=0  oneHot=off  pipeline_display=0  use_ena=off  use_aclr=off  allowFloatingPointOverride=on  logOutputs=off  logFile=C:\Users\ASUS\Desktop\sift_fpga\Octave_2\tb_test_final_sift\test%5Ffinal%5Fsift_sift%5Foctave1_get%5Fdescriptor_hist%5Fbin_Subsystem_Multiplexer3.fixedpointlog
  Multiplexer4 : allblocks_alteradspbuilder2/Multiplexer  numInputs=2  pipeline=0  oneHot=off  pipeline_display=0  use_ena=off  use_aclr=off  allowFloatingPointOverride=on  logOutputs=off  logFile=C:\Users\ASUS\Desktop\sift_fpga\Octave_2\tb_test_final_sift\test%5Ffinal%5Fsift_sift%5Foctave1_get%5Fdescriptor_hist%5Fbin_Subsystem_Multiplexer4.fixedpointlog
  Multiplexer5 : allblocks_alteradspbuilder2/Multiplexer  numInputs=2  pipeline=0  oneHot=off  pipeline_display=0  use_ena=off  use_aclr=off  allowFloatingPointOverride=on  logOutputs=off  logFile=C:\Users\ASUS\Desktop\sift_fpga\Octave_2\tb_test_final_sift\test%5Ffinal%5Fsift_sift%5Foctave1_get%5Fdescriptor_hist%5Fbin_Subsystem_Multiplexer5.fixedpointlog
  Multiplexer6 : allblocks_alteradspbuilder2/Multiplexer  numInputs=2  pipeline=0  oneHot=off  pipeline_display=0  use_ena=off  use_aclr=off  allowFloatingPointOverride=on  logOutputs=off  logFile=C:\Users\ASUS\Desktop\sift_fpga\Octave_2\tb_test_final_sift\test%5Ffinal%5Fsift_sift%5Foctave1_get%5Fdescriptor_hist%5Fbin_Subsystem_Multiplexer6.fixedpointlog
  Multiplexer7 : allblocks_alteradspbuilder2/Multiplexer  numInputs=2  pipeline=0  oneHot=off  pipeline_display=0  use_ena=off  use_aclr=off  allowFloatingPointOverride=on  logOutputs=off  logFile=C:\Users\ASUS\Desktop\sift_fpga\Octave_2\tb_test_final_sift\test%5Ffinal%5Fsift_sift%5Foctave1_get%5Fdescriptor_hist%5Fbin_Subsystem_Multiplexer7.fixedpointlog
  Multiplexer8 : allblocks_alteradspbuilder2/Multiplexer  numInputs=2  pipeline=0  oneHot=off  pipeline_display=0  use_ena=off  use_aclr=off  allowFloatingPointOverride=on  logOutputs=off  logFile=C:\Users\ASUS\Desktop\sift_fpga\Octave_2\tb_test_final_sift\test%5Ffinal%5Fsift_sift%5Foctave1_get%5Fdescriptor_hist%5Fbin_Subsystem_Multiplexer8.fixedpointlog
  Multiplexer9 : allblocks_alteradspbuilder2/Multiplexer  numInputs=2  pipeline=0  oneHot=off  pipeline_display=0  use_ena=off  use_aclr=off  allowFloatingPointOverride=on  logOutputs=off  logFile=C:\Users\ASUS\Desktop\sift_fpga\Octave_2\tb_test_final_sift\test%5Ffinal%5Fsift_sift%5Foctave1_get%5Fdescriptor_hist%5Fbin_Subsystem_Multiplexer9.fixedpointlog
  bin1_out : Outport
  bin2_out : Outport  Port=2
  bin3_out : Outport  Port=3
  bin4_out : Outport  Port=4
  bin5_out : Outport  Port=5
  bin6_out : Outport  Port=6
  bin7_out : Outport  Port=7
  bin8_out : Outport  Port=8
  wires:
  hist_in_bin1/1 -> [hist_in_bin1]
  hist_in_bin2/1 -> [hist_in_bin2]
  hist_in_bin3/1 -> [hist_in_bin3]
  hist_in_bin4/1 -> [hist_in_bin4]
  hist_in_bin5/1 -> [hist_in_bin5]
  hist_in_bin6/1 -> [hist_in_bin6]
  hist_in_bin7/1 -> [hist_in_bin7]
  hist_in_bin8/1 -> [hist_in_bin8]
  [hist_in_bin1] -> Comparator19/1
  [hist_in_bin2] -> Comparator19/2
  Comparator19/1 -> Multiplexer20/1
  [hist_in_bin1] -> Multiplexer20/2
  [hist_in_bin2] -> Multiplexer20/3
  Multiplexer20/1 -> Comparator4/1, Multiplexer4/2
  [hist_in_bin3] -> Comparator1/1
  [hist_in_bin4] -> Comparator1/2
  Comparator1/1 -> Multiplexer1/1
  [hist_in_bin3] -> Multiplexer1/2
  [hist_in_bin4] -> Multiplexer1/3
  Multiplexer1/1 -> Multiplexer4/3, Comparator4/2
  [hist_in_bin5] -> Comparator3/1
  [hist_in_bin6] -> Comparator3/2
  Comparator3/1 -> Multiplexer3/1
  [hist_in_bin5] -> Multiplexer3/2
  [hist_in_bin6] -> Multiplexer3/3
  Multiplexer3/1 -> Comparator5/1, Multiplexer5/2
  [hist_in_bin7] -> Comparator2/1
  [hist_in_bin8] -> Comparator2/2
  Comparator2/1 -> Multiplexer2/1
  [hist_in_bin7] -> Multiplexer2/2
  [hist_in_bin8] -> Multiplexer2/3
  Multiplexer2/1 -> Multiplexer5/3, Comparator5/2
  Comparator4/1 -> Multiplexer4/1
  Comparator5/1 -> Multiplexer5/1
  Multiplexer4/1 -> Multiplexer6/2, Comparator6/1
  Multiplexer5/1 -> Comparator6/2, Multiplexer6/3
  Comparator6/1 -> Multiplexer6/1
  Multiplexer6/1 -> Logical Bus Operator/1
  Logical Bus Operator/1 -> [threshold]
  [hist_in_bin1] -> Comparator8/1
  [threshold] -> Comparator8/2
  Comparator8/1 -> Multiplexer9/1
  [hist_in_bin1] -> Multiplexer9/2
  [hist_in_bin2] -> Comparator7/1
  [threshold] -> Comparator7/2
  Comparator7/1 -> Multiplexer7/1
  [hist_in_bin2] -> Multiplexer7/2
  [hist_in_bin3] -> Comparator10/1
  [threshold] -> Comparator10/2
  Comparator10/1 -> Multiplexer10/1
  [hist_in_bin3] -> Multiplexer10/2
  [hist_in_bin4] -> Comparator9/1
  [threshold] -> Comparator9/2
  Comparator9/1 -> Multiplexer8/1
  [hist_in_bin4] -> Multiplexer8/2
  [hist_in_bin5] -> Comparator12/1
  [threshold] -> Comparator12/2
  Comparator12/1 -> Multiplexer13/1
  [hist_in_bin5] -> Multiplexer13/2
  [hist_in_bin6] -> Comparator11/1
  [threshold] -> Comparator11/2
  Comparator11/1 -> Multiplexer11/1
  [hist_in_bin6] -> Multiplexer11/2
  [hist_in_bin7] -> Comparator14/1
  [threshold] -> Comparator14/2
  Comparator14/1 -> Multiplexer14/1
  [hist_in_bin7] -> Multiplexer14/2
  [hist_in_bin8] -> Comparator13/1
  [threshold] -> Comparator13/2
  Comparator13/1 -> Multiplexer12/1
  [hist_in_bin8] -> Multiplexer12/2
  Multiplexer9/1 -> bin1_out/1
  Multiplexer7/1 -> bin2_out/1
  Multiplexer10/1 -> bin3_out/1
  Multiplexer8/1 -> bin4_out/1
  Multiplexer13/1 -> bin5_out/1
  Multiplexer11/1 -> bin6_out/1
  Multiplexer14/1 -> bin7_out/1
  Multiplexer12/1 -> bin8_out/1
  Constant/1 -> Multiplexer9/3
  Constant1/1 -> Multiplexer7/3
  Constant2/1 -> Multiplexer10/3
  Constant3/1 -> Multiplexer8/3
  Constant4/1 -> Multiplexer12/3
  Constant5/1 -> Multiplexer14/3
  Constant6/1 -> Multiplexer11/3
  Constant7/1 -> Multiplexer13/3
